simulink model "Longitudinaldynamicmodel_SmartFortwo"  (R2021b)
settings: Solver=FixedStepAuto  StartTime=0.0  StopTime=1  FixedStep=0.01  RelTol=1e-3
undefined symbols (not defined in the file): DiscIntNeverNeededParam, VehMass
libraries: Constant_Environment x1, Driver_PI x1, Longitudinal_DrivingCycles x1, Acceleration_Calculation x1, Air_Resistance x1, Roll_Resistance x1, Slope_Resistance x1, Constant_Power_Source x1, Simple_Auxiliary x1, Electric_Drive_Tabled_Consumption x1, Gear_Stage x1, DCAC_Converter x1
(part 3 of 3)

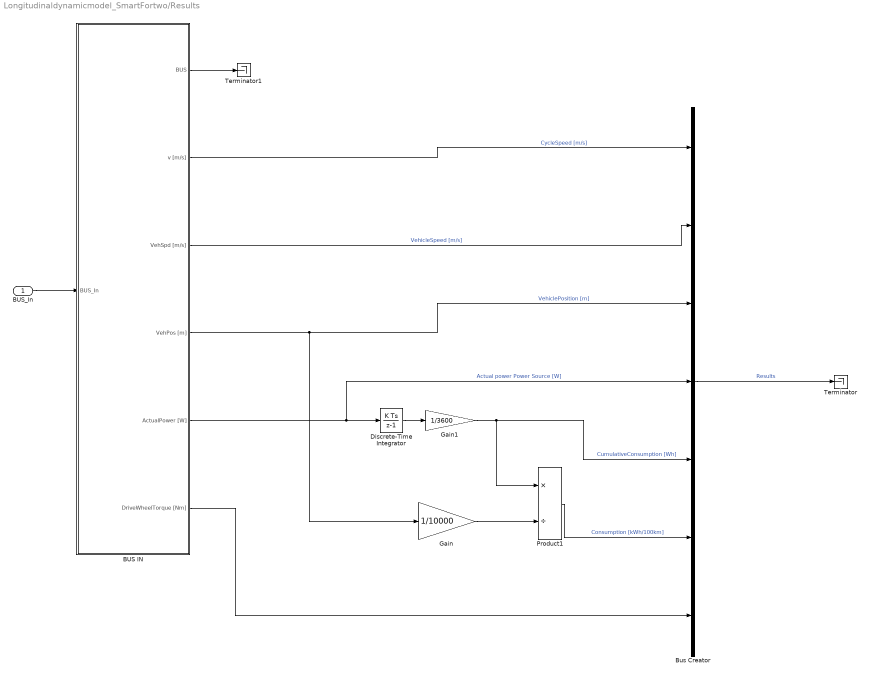
== system Longitudinaldynamicmodel_SmartFortwo/Results ==
  BUS_In : Inport
  BUS IN : Subsystem
      mask help:
      | <Author> Alexander Koch
      | <Date> 02/05/2017
      | <Predecessor> Stefan Müller, Stephan Rohr
      |
      | <Description>
      | Automated BUS IN Block for the Bus System. After the Bus In is connected and receives signals it is possible to choose the required signals by clicking on the block. After choosing the signals it is possible to push the Refresh button. This button builds the required amount of outputs, connects the Bus Selector and the Outputs and rename all the outputs with the corresponding signal name.
      |
      | The Block automaticlly disconnects the link to the library block after opening the first time
      |
      | <Parameters>
      | -
      |
      | <Inputs>
      | Bus [Bus]
      |
      | <Outputs>
      | Bus [Bus]
      | SignalName[-]
      mask init:
      | BusInInitFct()
      settings: OpenFcn=|
      | set_param(gcb(),'LinkStatus','none')
      | open_system(gcb(),'mask')
      | open_system(strcat(gcb(),'/Bus Selector'),'Parameter')
      mask DialogControl ParameterGroupVar Prompt: Refresh
      mask DialogControl RefreshOutputs Prompt: Refresh all Output Names
      mask DialogControl RefreshOutputs Callback: BusInInitFct()
  Bus Creator : BusCreator  Inputs=7
  Discrete-Time Integrator : DiscreteIntegrator  SampleTime=-1  ICPrevOutput=DiscIntNeverNeededParam  ICPrevScaledInput=DiscIntNeverNeededParam
  Gain : Gain  Gain=1/10000
  Gain1 : Gain  Gain=1/3600
  Product1 : Product  Inputs=*/
  Terminator : Terminator
  Terminator1 : Terminator
  wires:
  BUS_In/1 -> BUS IN/1(BUS_In)
  BUS IN/1(BUS) -> Terminator1/1
  Bus Creator/1 -> Terminator/1  "Results"
  Discrete-Time Integrator/1 -> Gain1/1
  Gain1/1 -> Bus Creator/5, Product1/1  "CumulativeConsumption [Wh]"
  BUS IN/5(ActualPower [W]) -> Bus Creator/4, Discrete-Time Integrator/1  "Actual power Power Source [W]"
  BUS IN/2(v [m/s]) -> Bus Creator/1  "CycleSpeed [m/s]"
  BUS IN/3(VehSpd [m/s]) -> Bus Creator/2  "VehicleSpeed [m/s]"
  BUS IN/4(VehPos [m]) -> Bus Creator/3, Gain/1  "VehiclePosition [m]"
  BUS IN/6(DriveWheelTorque [Nm]) -> Bus Creator/7
  Gain/1 -> Product1/2
  Product1/1 -> Bus Creator/6  "Consumption [kWh/100km]"

== system Longitudinaldynamicmodel_SmartFortwo/Timer and Bus Reset ==
  BUS_In : Inport
  Bus Creator : BusCreator  Inputs=1
  Bus Selector : BusSelector  OutputSignals=Dynamics,Powertrain,Powersource,VehicleControlUnit,Driver and Environment,DrivinCycle  OutputAsBus=on
  Unit Delay : UnitDelay  SampleTime=-1  HasFrameUpgradeWarning=on
  BUS_Out : Outport  VectorParamsAs1DForOutWhenUnconnected=off
  wires:
  Bus Creator/1 -> BUS_Out/1
  Bus Selector/1 -> Unit Delay/1
  Unit Delay/1 -> Bus Creator/1  "Bus_Old"
  BUS_In/1 -> Bus Selector/1

== system Longitudinaldynamicmodel_SmartFortwo/Vehicle Control Unit ==
  BUS_In : Inport
  BUS IN : Subsystem
      mask help:
      | <Author> Alexander Koch based on Stefan Müller, Stephan Rohr
      | <Date> 02/05/2017
      |
      | <Description>
      | Automated BUS IN Block for the Bus System. After the Bus In is connected and receives signals it is possible to choose the required signals by clicking on the block. After choosing the signals it is possible to push the Refresh button. This button builds the required amount of outputs, connects the Bus Selector and the Outputs and rename all the outputs with the corresponding signal name.
      |
      | The Block automaticlly disconnects the link to the library block after opening the first time
      |
      | <Parameters>
      | -
      |
      | <Inputs>
      | Bus [Bus]
      |
      | <Outputs>
      | Bus [Bus]
      | SignalName[-]
      mask init:
      | BusInInitFct()
      settings: OpenFcn=|
      | set_param(gcb(),'LinkStatus','none')
      | open_system(gcb(),'mask')
      | open_system(strcat(gcb(),'/Bus Selector'),'Parameter')
      mask DialogControl ParameterGroupVar Prompt: Refresh
      mask DialogControl RefreshOutputs Prompt: Refresh all Output Names
      mask DialogControl RefreshOutputs Callback: BusInInitFct()
  BUS OUT : Subsystem  mask{NumberofInputs=3, NameSys='VehicleControlUnit'}
      mask prompts: NumberofInputs "Numper of costum inputs"; NameSys "Name of Bus Subsystem"
      mask help:
      | <Author> Alexander Koch based on Stefan Müller, Stephan Rohr
      | <Date> 02/05/2017
      |
      | <Description>
      | Automated BUS Out Block for the Bus System. Allows to enter the Number of costum inputs and the name of the bus system. After entering the parameters the required amout of Inputs are built and connected to the Bus Creator. The signal names that are connected to the inputs In1, ..., InN are automatically adopted at the Bus signal names and can be found in the Bus under the name of the Bus Subsystem. If the signal (line) to the Inport has no name, the name of the previous blocks outport is taken. If this is not possible, the name if the previous block is taken for the Bus signal name.
      |
      | Additional, there are two buttons. The Refresh Input Names refreshes all Input Names. This is required if signal names are changed or signals are connected for the first time. To build a new system or if another Subsystem is added between existing subsystems, the Refresh Bus Selector is required at every subsystem that is calculated after the new subsystem.
      |
      | The Block automaticlly disconnects the link to the library block after opening the first time
      |
      | <Parameters>
      | Number of costum inputs [-]
      | Name of Bus Subsystem ['abc']
      |
      | <Inputs>
      | Bus [Bus]
      | In1 [ ]
      |
      | <Outputs>
      | Bus [Bus]
      mask init:
      | BusRefreshInputs()
      settings: OpenFcn=|
      | set_param(gcb(),'LinkStatus','none')
      | open_system(gcb(),'mask')
      mask DialogControl Container3 Prompt: Refresh
      mask DialogControl RefreshInputNames Prompt: Refresh Input Names
      mask DialogControl RefreshInputNames Callback: BusRefreshLineNames()
      mask DialogControl RefreshBusSelector Prompt: Refresh Bus Selector
      mask DialogControl RefreshBusSelector Callback: BusRefreshBusSelector()
  Control Unit Simple : Control_Unit_Simple/Control Unit Simple  Brake_Distribution_Front=0.7  MaxBrkTrq=448  MaxMotorTrq=110  LocalSampleTime=0.01
  BUS_Out : Outport  VectorParamsAs1DForOutWhenUnconnected=off
  wires:
  BUS IN/1(BUS) -> BUS OUT/1(BUS)
  BUS OUT/1(BUS_OUT) -> BUS_Out/1
  BUS_In/1 -> BUS IN/1(BUS_In)
  Control Unit Simple/2 -> BUS OUT/3(In2)
  Control Unit Simple/3 -> BUS OUT/4(In3)
  Control Unit Simple/1 -> BUS OUT/2(In1)
  BUS IN/2(AccPedalPos [-]) -> Control Unit Simple/1
  BUS IN/3(BrakePedalPos [-]) -> Control Unit Simple/2

== system Longitudinaldynamicmodel_SmartFortwo/Driver and Environment/BUS IN ==
  BUS_In : Inport
  Bus Selector : BusSelector  OutputSignals=DrivinCycle.v [m/s],Bus_Old.Dynamics.VehSpd [m/s]
  BUS : Outport  VectorParamsAs1DForOutWhenUnconnected=off
  v [m/s] : Outport  Port=2  VectorParamsAs1DForOutWhenUnconnected=off
  VehSpd [m/s] : Outport  Port=3  VectorParamsAs1DForOutWhenUnconnected=off
  wires:
  BUS_In/1 -> Bus Selector/1, BUS/1
  Bus Selector/1 -> v [m/s]/1  "<v [m/s]>"
  Bus Selector/2 -> VehSpd [m/s]/1  "<VehSpd [m/s]>"

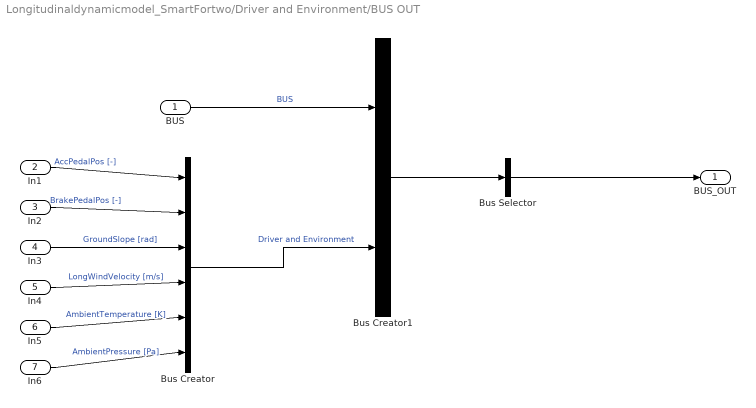
== system Longitudinaldynamicmodel_SmartFortwo/Driver and Environment/BUS OUT ==
  BUS : Inport
  In1 : Inport  Port=2
  In2 : Inport  Port=3
  In3 : Inport  Port=4
  In4 : Inport  Port=5
  In5 : Inport  Port=6
  In6 : Inport  Port=7
  Bus Creator : BusCreator  Inputs=6
  Bus Creator1 : BusCreator  Inputs=2
  Bus Selector : BusSelector  OutputSignals=Driver and Environment,BUS.DrivinCycle,BUS.Bus_Old  OutputAsBus=on
  BUS_OUT : Outport  VectorParamsAs1DForOutWhenUnconnected=off
  wires:
  Bus Creator1/1 -> Bus Selector/1
  BUS/1 -> Bus Creator1/1  "BUS"
  Bus Creator/1 -> Bus Creator1/2  "Driver and Environment"
  Bus Selector/1 -> BUS_OUT/1
  In1/1 -> Bus Creator/1  "AccPedalPos [-]"
  In2/1 -> Bus Creator/2  "BrakePedalPos [-]"
  In3/1 -> Bus Creator/3  "GroundSlope [rad]"
  In4/1 -> Bus Creator/4  "LongWindVelocity [m/s]"
  In5/1 -> Bus Creator/5  "AmbientTemperature [K]"
  In6/1 -> Bus Creator/6  "AmbientPressure [Pa]"

== system Longitudinaldynamicmodel_SmartFortwo/Driving Cycle/BUS IN ==
  BUS_In : Inport
  Bus Selector : BusSelector  OutputSignals=Bus_Old.Dynamics.VehSpd [m/s]
  BUS : Outport  VectorParamsAs1DForOutWhenUnconnected=off
  VehSpd [m/s] : Outport  Port=2  VectorParamsAs1DForOutWhenUnconnected=off
  wires:
  BUS_In/1 -> Bus Selector/1, BUS/1
  Bus Selector/1 -> VehSpd [m/s]/1  "<VehSpd [m/s]>"

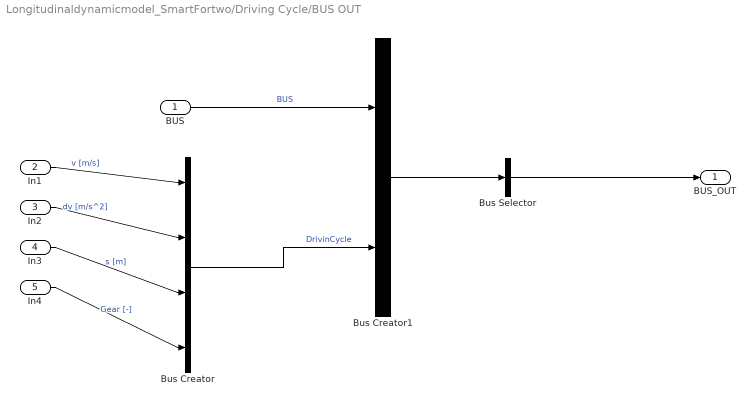
== system Longitudinaldynamicmodel_SmartFortwo/Driving Cycle/BUS OUT ==
  BUS : Inport
  In1 : Inport  Port=2
  In2 : Inport  Port=3
  In3 : Inport  Port=4
  In4 : Inport  Port=5
  Bus Creator : BusCreator  Inputs=4
  Bus Creator1 : BusCreator  Inputs=2
  Bus Selector : BusSelector  OutputSignals=DrivinCycle,BUS.Bus_Old  OutputAsBus=on
  BUS_OUT : Outport  VectorParamsAs1DForOutWhenUnconnected=off
  wires:
  Bus Creator1/1 -> Bus Selector/1
  BUS/1 -> Bus Creator1/1  "BUS"
  Bus Creator/1 -> Bus Creator1/2  "DrivinCycle"
  Bus Selector/1 -> BUS_OUT/1
  In1/1 -> Bus Creator/1  "v [m/s]"
  In2/1 -> Bus Creator/2  "dv [m/s^2]"
  In3/1 -> Bus Creator/3  "s [m]"
  In4/1 -> Bus Creator/4  "Gear [-]"

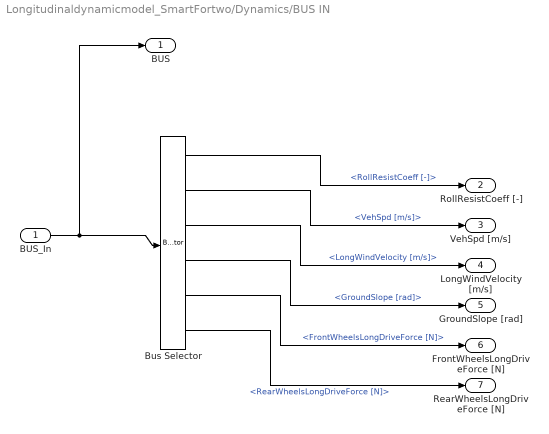
== system Longitudinaldynamicmodel_SmartFortwo/Dynamics/BUS IN ==
  BUS_In : Inport
  Bus Selector : BusSelector  OutputSignals=Powertrain.RollResistCoeff [-],Bus_Old.Dynamics.VehSpd [m/s],Driver and Environment.LongWindVelocity [m/s],Driver and Environment.GroundSlope [rad],Powertrain.FrontWheelsLongDriveForce [N],Powertrain.RearWheelsLongDriveForce [N]
  BUS : Outport  VectorParamsAs1DForOutWhenUnconnected=off
  RollResistCoeff [-] : Outport  Port=2  VectorParamsAs1DForOutWhenUnconnected=off
  VehSpd [m/s] : Outport  Port=3  VectorParamsAs1DForOutWhenUnconnected=off
  LongWindVelocity [m/s] : Outport  Port=4  VectorParamsAs1DForOutWhenUnconnected=off
  GroundSlope [rad] : Outport  Port=5  VectorParamsAs1DForOutWhenUnconnected=off
  FrontWheelsLongDriveForce [N] : Outport  Port=6  VectorParamsAs1DForOutWhenUnconnected=off
  RearWheelsLongDriveForce [N] : Outport  Port=7  VectorParamsAs1DForOutWhenUnconnected=off
  wires:
  BUS_In/1 -> Bus Selector/1, BUS/1
  Bus Selector/1 -> RollResistCoeff [-]/1  "<RollResistCoeff [-]>"
  Bus Selector/2 -> VehSpd [m/s]/1  "<VehSpd [m/s]>"
  Bus Selector/3 -> LongWindVelocity [m/s]/1  "<LongWindVelocity [m/s]>"
  Bus Selector/4 -> GroundSlope [rad]/1  "<GroundSlope [rad]>"
  Bus Selector/5 -> FrontWheelsLongDriveForce [N]/1  "<FrontWheelsLongDriveForce [N]>"
  Bus Selector/6 -> RearWheelsLongDriveForce [N]/1  "<RearWheelsLongDriveForce [N]>"

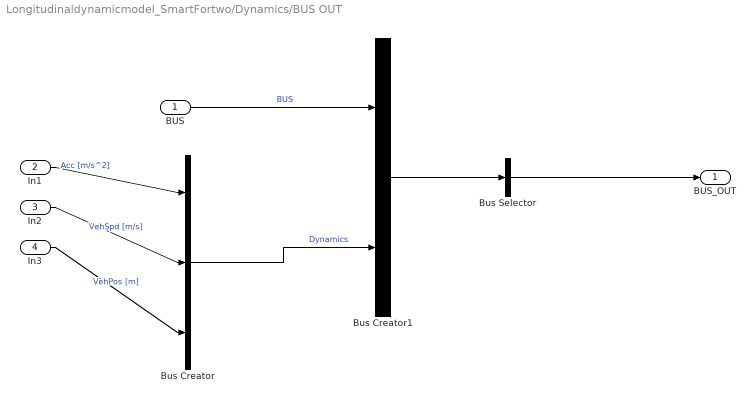
== system Longitudinaldynamicmodel_SmartFortwo/Dynamics/BUS OUT ==
  BUS : Inport
  In1 : Inport  Port=2
  In2 : Inport  Port=3
  In3 : Inport  Port=4
  Bus Creator : BusCreator  Inputs=3
  Bus Creator1 : BusCreator  Inputs=2
  Bus Selector : BusSelector  OutputSignals=Dynamics,BUS.Powertrain,BUS.Powersource,BUS.VehicleControlUnit,BUS.Driver and Environment,BUS.DrivinCycle,BUS.Bus_Old  OutputAsBus=on
  BUS_OUT : Outport  VectorParamsAs1DForOutWhenUnconnected=off
  wires:
  Bus Creator1/1 -> Bus Selector/1
  BUS/1 -> Bus Creator1/1  "BUS"
  Bus Creator/1 -> Bus Creator1/2  "Dynamics"
  Bus Selector/1 -> BUS_OUT/1
  In1/1 -> Bus Creator/1  "Acc [m/s^2]"
  In2/1 -> Bus Creator/2  "VehSpd [m/s]"
  In3/1 -> Bus Creator/3  "VehPos [m]"

== system Longitudinaldynamicmodel_SmartFortwo/Power Source/BUS IN ==
  BUS_In : Inport
  Bus Selector : BusSelector  OutputSignals=Bus_Old.Powertrain.PowertrainPowerReq [W]
  BUS : Outport  VectorParamsAs1DForOutWhenUnconnected=off
  PowertrainPowerReq [W] : Outport  Port=2  VectorParamsAs1DForOutWhenUnconnected=off
  wires:
  BUS_In/1 -> Bus Selector/1, BUS/1
  Bus Selector/1 -> PowertrainPowerReq [W]/1  "<PowertrainPowerReq [W]>"

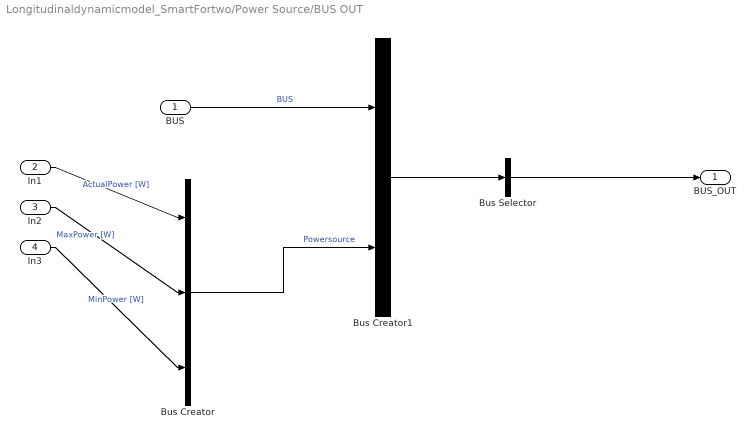
== system Longitudinaldynamicmodel_SmartFortwo/Power Source/BUS OUT ==
  BUS : Inport
  In1 : Inport  Port=2
  In2 : Inport  Port=3
  In3 : Inport  Port=4
  Bus Creator : BusCreator  Inputs=3
  Bus Creator1 : BusCreator  Inputs=2
  Bus Selector : BusSelector  OutputSignals=Powersource,BUS.VehicleControlUnit,BUS.Driver and Environment,BUS.DrivinCycle,BUS.Bus_Old  OutputAsBus=on
  BUS_OUT : Outport  VectorParamsAs1DForOutWhenUnconnected=off
  wires:
  Bus Creator1/1 -> Bus Selector/1
  BUS/1 -> Bus Creator1/1  "BUS"
  Bus Creator/1 -> Bus Creator1/2  "Powersource"
  Bus Selector/1 -> BUS_OUT/1
  In1/1 -> Bus Creator/1  "ActualPower [W]"
  In2/1 -> Bus Creator/2  "MaxPower [W]"
  In3/1 -> Bus Creator/3  "MinPower [W]"

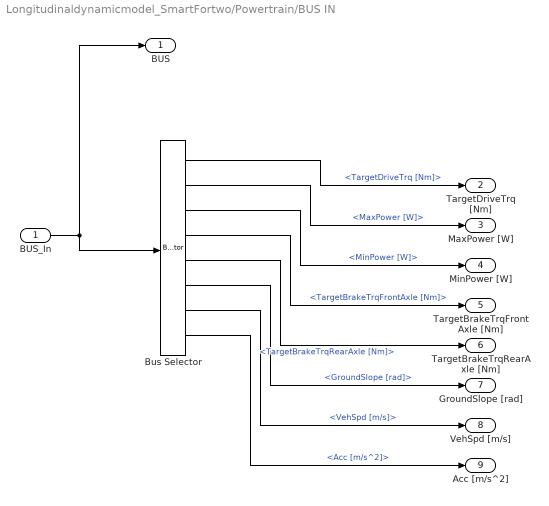
== system Longitudinaldynamicmodel_SmartFortwo/Powertrain/BUS IN ==
  BUS_In : Inport
  Bus Selector : BusSelector  OutputSignals=VehicleControlUnit.TargetDriveTrq [Nm],Powersource.MaxPower [W],Powersource.MinPower [W],VehicleControlUnit.TargetBrakeTrqFrontAxle [Nm],VehicleControlUnit.TargetBrakeTrqRearAxle [Nm],Driver and Environment.GroundSlope [rad],Bus_Old.Dynamics.VehSpd [m/s],Bus_Old.Dynamics.Acc [m/s^2]
  BUS : Outport  VectorParamsAs1DForOutWhenUnconnected=off
  TargetDriveTrq [Nm] : Outport  Port=2  VectorParamsAs1DForOutWhenUnconnected=off
  MaxPower [W] : Outport  Port=3  VectorParamsAs1DForOutWhenUnconnected=off
  MinPower [W] : Outport  Port=4  VectorParamsAs1DForOutWhenUnconnected=off
  TargetBrakeTrqFrontAxle [Nm] : Outport  Port=5  VectorParamsAs1DForOutWhenUnconnected=off
  TargetBrakeTrqRearAxle [Nm] : Outport  Port=6  VectorParamsAs1DForOutWhenUnconnected=off
  GroundSlope [rad] : Outport  Port=7  VectorParamsAs1DForOutWhenUnconnected=off
  VehSpd [m/s] : Outport  Port=8  VectorParamsAs1DForOutWhenUnconnected=off
  Acc [m/s^2] : Outport  Port=9  VectorParamsAs1DForOutWhenUnconnected=off
  wires:
  BUS_In/1 -> Bus Selector/1, BUS/1
  Bus Selector/1 -> TargetDriveTrq [Nm]/1  "<TargetDriveTrq [Nm]>"
  Bus Selector/2 -> MaxPower [W]/1  "<MaxPower [W]>"
  Bus Selector/3 -> MinPower [W]/1  "<MinPower [W]>"
  Bus Selector/4 -> TargetBrakeTrqFrontAxle [Nm]/1  "<TargetBrakeTrqFrontAxle [Nm]>"
  Bus Selector/5 -> TargetBrakeTrqRearAxle [Nm]/1  "<TargetBrakeTrqRearAxle [Nm]>"
  Bus Selector/6 -> GroundSlope [rad]/1  "<GroundSlope [rad]>"
  Bus Selector/7 -> VehSpd [m/s]/1  "<VehSpd [m/s]>"
  Bus Selector/8 -> Acc [m/s^2]/1  "<Acc [m/s^2]>"

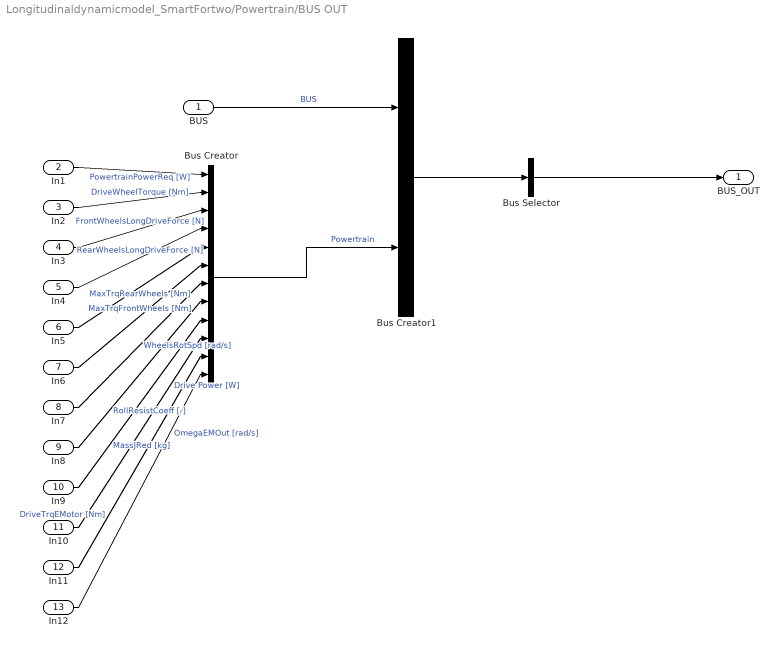
== system Longitudinaldynamicmodel_SmartFortwo/Powertrain/BUS OUT ==
  BUS : Inport
  In1 : Inport  Port=2
  In2 : Inport  Port=3
  In3 : Inport  Port=4
  In4 : Inport  Port=5
  In5 : Inport  Port=6
  In6 : Inport  Port=7
  In7 : Inport  Port=8
  In8 : Inport  Port=9
  In9 : Inport  Port=10
  In10 : Inport  Port=11
  In11 : Inport  Port=12
  In12 : Inport  Port=13
  Bus Creator : BusCreator  Inputs=12
  Bus Creator1 : BusCreator  Inputs=2
  Bus Selector : BusSelector  OutputSignals=Powertrain,BUS.Powersource,BUS.VehicleControlUnit,BUS.Driver and Environment,BUS.DrivinCycle,BUS.Bus_Old  OutputAsBus=on
  BUS_OUT : Outport  VectorParamsAs1DForOutWhenUnconnected=off
  wires:
  Bus Creator1/1 -> Bus Selector/1
  BUS/1 -> Bus Creator1/1  "BUS"
  Bus Creator/1 -> Bus Creator1/2  "Powertrain"
  Bus Selector/1 -> BUS_OUT/1
  In1/1 -> Bus Creator/1  "PowertrainPowerReq [W]"
  In2/1 -> Bus Creator/2  "DriveWheelTorque [Nm]"
  In3/1 -> Bus Creator/3  "FrontWheelsLongDriveForce [N]"
  In4/1 -> Bus Creator/4  "RearWheelsLongDriveForce [N]"
  In5/1 -> Bus Creator/5  "MaxTrqRearWheels [Nm]"
  In6/1 -> Bus Creator/6  "MaxTrqFrontWheels [Nm]"
  In7/1 -> Bus Creator/7  "WheelsRotSpd [rad/s]"
  In8/1 -> Bus Creator/8  "RollResistCoeff [-]"
  In9/1 -> Bus Creator/9  "MassJRed [kg]"
  In10/1 -> Bus Creator/10  "Drive Power [W]"
  In11/1 -> Bus Creator/11  "DriveTrqEMotor [Nm]"
  In12/1 -> Bus Creator/12  "OmegaEMOut [rad/s]"

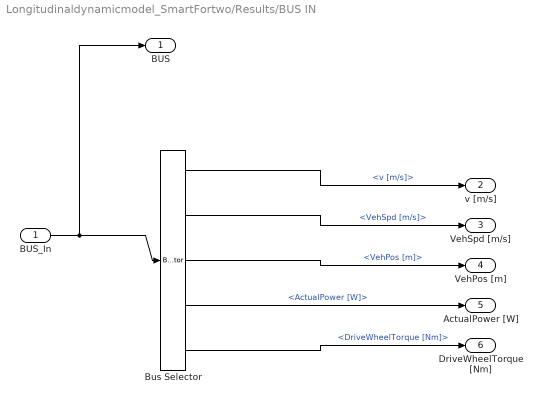
== system Longitudinaldynamicmodel_SmartFortwo/Results/BUS IN ==
  BUS_In : Inport
  Bus Selector : BusSelector  OutputSignals=DrivinCycle.v [m/s],Dynamics.VehSpd [m/s],Dynamics.VehPos [m],Powersource.ActualPower [W],Powertrain.DriveWheelTorque [Nm]
  BUS : Outport  VectorParamsAs1DForOutWhenUnconnected=off
  v [m/s] : Outport  Port=2  VectorParamsAs1DForOutWhenUnconnected=off
  VehSpd [m/s] : Outport  Port=3  VectorParamsAs1DForOutWhenUnconnected=off
  VehPos [m] : Outport  Port=4  VectorParamsAs1DForOutWhenUnconnected=off
  ActualPower [W] : Outport  Port=5  VectorParamsAs1DForOutWhenUnconnected=off
  DriveWheelTorque [Nm] : Outport  Port=6  VectorParamsAs1DForOutWhenUnconnected=off
  wires:
  BUS_In/1 -> BUS/1, Bus Selector/1
  Bus Selector/1 -> v [m/s]/1  "<v [m/s]>"
  Bus Selector/2 -> VehSpd [m/s]/1  "<VehSpd [m/s]>"
  Bus Selector/3 -> VehPos [m]/1  "<VehPos [m]>"
  Bus Selector/4 -> ActualPower [W]/1  "<ActualPower [W]>"
  Bus Selector/5 -> DriveWheelTorque [Nm]/1  "<DriveWheelTorque [Nm]>"

== system Longitudinaldynamicmodel_SmartFortwo/Vehicle Control Unit/BUS IN ==
  BUS_In : Inport
  Bus Selector : BusSelector  OutputSignals=Driver and Environment.AccPedalPos [-],Driver and Environment.BrakePedalPos [-]
  BUS : Outport  VectorParamsAs1DForOutWhenUnconnected=off
  AccPedalPos [-] : Outport  Port=2  VectorParamsAs1DForOutWhenUnconnected=off
  BrakePedalPos [-] : Outport  Port=3  VectorParamsAs1DForOutWhenUnconnected=off
  wires:
  BUS_In/1 -> Bus Selector/1, BUS/1
  Bus Selector/1 -> AccPedalPos [-]/1  "<AccPedalPos [-]>"
  Bus Selector/2 -> BrakePedalPos [-]/1  "<BrakePedalPos [-]>"

== system Longitudinaldynamicmodel_SmartFortwo/Vehicle Control Unit/BUS OUT ==
  BUS : Inport
  In1 : Inport  Port=2
  In2 : Inport  Port=3
  In3 : Inport  Port=4
  Bus Creator : BusCreator  Inputs=3
  Bus Creator1 : BusCreator  Inputs=2
  Bus Selector : BusSelector  OutputSignals=VehicleControlUnit,BUS.Driver and Environment,BUS.DrivinCycle,BUS.Bus_Old  OutputAsBus=on
  BUS_OUT : Outport  VectorParamsAs1DForOutWhenUnconnected=off
  wires:
  Bus Creator1/1 -> Bus Selector/1
  BUS/1 -> Bus Creator1/1  "BUS"
  Bus Creator/1 -> Bus Creator1/2  "VehicleControlUnit"
  Bus Selector/1 -> BUS_OUT/1
  In1/1 -> Bus Creator/1  "TargetDriveTrq [Nm]"
  In2/1 -> Bus Creator/2  "TargetBrakeTrqFrontAxle [Nm]"
  In3/1 -> Bus Creator/3  "TargetBrakeTrqRearAxle [Nm]"
